simulink model "LBMPC"  (R2018b)
settings: Solver=VariableStepAuto  StartTime=0.0  StopTime=10  RelTol=1e-3
values from neighbouring files (symbols this model uses):
  Ad = expm(A*dT)    [init_ctrl_design.m]    (also in init_ctrl_design_simple.m = eye(2)+A*Ts)
  Bd = (Ad-eye(n))*inv(A)*B    [init_ctrl_design.m]    (also in init_ctrl_design_simple.m = Ts*B)
  beta = 1    [TaylorRemainder.m]    (also in init_ctrl_design.m; init_ctrl_design_simple.m; solveMGCM.m)
  Cd = C    [init_ctrl_design.m]    (also in init_ctrl_design_simple.m = eye(2))
  Dd = D    [init_ctrl_design.m]    (also in init_ctrl_design_simple.m)
  init_cond = [x1-0.35, x2-0.4, x3, 0]    [TaylorRemainder.m]    (also in init_ctrl_design.m; init_ctrl_design_simple.m = [x1-0.35, x2-0.4])
  Ts = 0.01    [APRBSgeneration.m]    (also in draw.m; drawCP.m = 0.1; genTrainingData.m = 0.1; init_ctrl_design.m)
  wn = sqrt(1000)    [TaylorRemainder.m]    (also in init_ctrl_design.m; solveMGCM.m)
  x2_c = 0    [TaylorRemainder.m]    (also in init_ctrl_design.m; init_ctrl_design_simple.m; solveMGCM.m)
  zeta = 1/sqrt(2)    [TaylorRemainder.m]    (also in init_ctrl_design.m)
undefined symbols (not defined in the file or in its folder): DiscIntNeverNeededParam, K
settings Model: Creator=pbevanda  LastModifiedBy=pbevanda

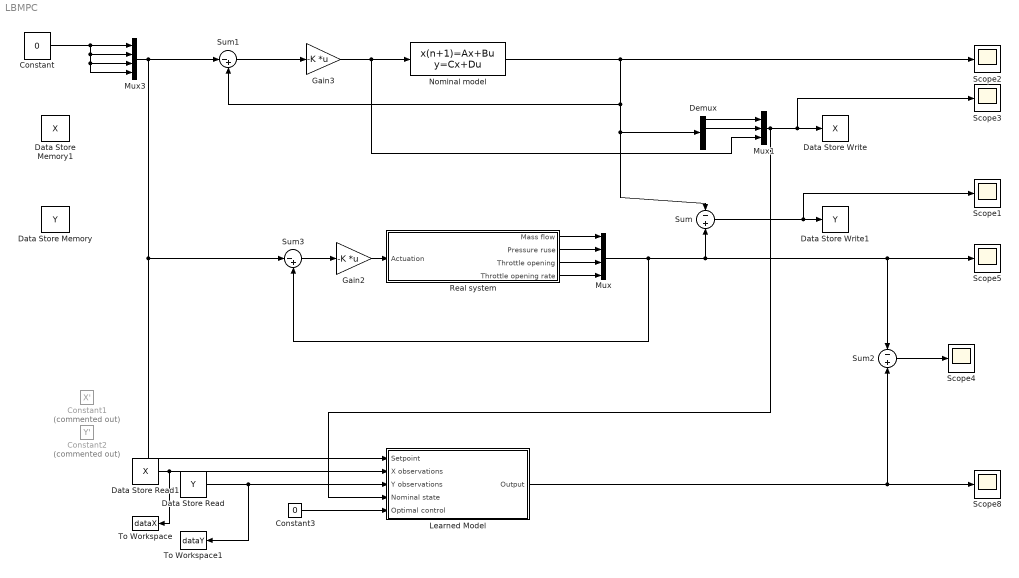
== system LBMPC ==
  "  Nominal model" : DiscreteStateSpace  A=Ad  B=Bd  C=Cd  D=Dd  InitialCondition=init_cond  SampleTime=Ts
  Constant : Constant  Value=0
  Constant1 : Constant  Commented=on  Value=X'  VectorParams1D=off  SampleTime=1
  Constant2 : Constant  Commented=on  Value=Y'  VectorParams1D=off
  Constant3 : Constant  Value=0  VectorParams1D=off
  Data Store Memory : DataStoreMemory  DataStoreName=Y  ReadBeforeWriteMsg=warning  WriteAfterWriteMsg=warning  WriteAfterReadMsg=warning  ShowAdditionalParam=off  OutDataTypeStr=double  Dimensions=4
  Data Store Memory1 : DataStoreMemory  DataStoreName=X  ReadBeforeWriteMsg=warning  WriteAfterWriteMsg=warning  WriteAfterReadMsg=warning  ShowAdditionalParam=off  OutDataTypeStr=double  Dimensions=3
  Data Store Read : DataStoreRead  DataStoreName=Y
  Data Store Read1 : DataStoreRead  DataStoreName=X
  Data Store Write : DataStoreWrite  DataStoreName=X
  Data Store Write1 : DataStoreWrite  DataStoreName=Y
  Demux : Demux
  Gain2 : Gain  Gain=-K  Multiplication=Matrix(K*u)
  Gain3 : Gain  Gain=-K  Multiplication=Matrix(K*u)
  "Learned Model " : Subsystem
  Mux : Mux
  Mux1 : Mux  Inputs=3
  Mux3 : Mux
  Real system : Subsystem
  Scope{1..5,8} (6 alike) : Scope
  Sum : Sum  Inputs=-+
  Sum1 : Sum  Inputs=|-+
  Sum2 : Sum  Inputs=-+
  Sum3 : Sum  Inputs=|-+
  To Workspace : ToWorkspace  VariableName=dataX  SampleTime=-1
  To Workspace1 : ToWorkspace  VariableName=dataY  SampleTime=-1
  wires:
  Gain2/1 -> Real system/1("Actuation ")
  Sum1/1 -> Gain3/1
  Demux/1 -> Mux1/1
  Real system/1("Mass flow ") -> Mux/1
  "  Nominal model"/1 -> Demux/1, Sum/1, Sum1/2, Scope2/1
  Constant/1 -> Mux3/1, Mux3/4, Mux3/3, Mux3/2
  Mux/1 -> Sum3/2, Sum2/1, Scope5/1, Sum/2
  Sum3/1 -> Gain2/1
  Real system/4("Throttle opening rate ") -> Mux/4
  Demux/2 -> Mux1/2
  Mux3/1 -> Sum1/1, "Learned Model "/1(Setpoint), Sum3/1
  Real system/2("Pressure ruse ") -> Mux/2
  Gain3/1 -> "  Nominal model"/1, Mux1/3
  Real system/3("Throttle opening ") -> Mux/3
  Sum/1 -> Scope1/1, Data Store Write1/1
  Constant3/1 -> "Learned Model "/5(Optimal control)
  "Learned Model "/1("Output ") -> Sum2/2, Scope8/1
  Mux1/1 -> "Learned Model "/4(Nominal state), Scope3/1, Data Store Write/1
  Data Store Read/1 -> To Workspace1/1, "Learned Model "/3(Y observations)
  Data Store Read1/1 -> To Workspace/1, "Learned Model "/2("X observations ")
  Sum2/1 -> Scope4/1

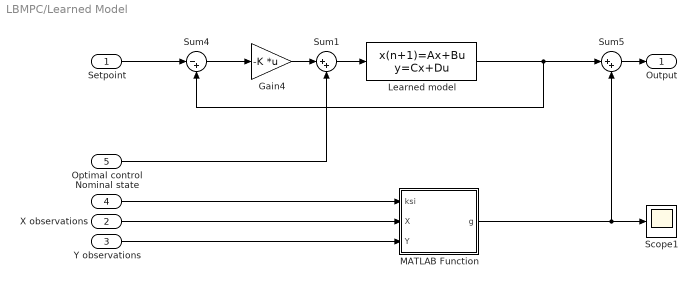
== system LBMPC/Learned Model  ==
  Setpoint : Inport
  "X observations " : Inport  Port=2
  Y observations : Inport  Port=3
  Nominal state : Inport  Port=4
  Optimal control : Inport  Port=5
  Gain4 : Gain  Gain=-K  Multiplication=Matrix(K*u)
  Learned model : DiscreteStateSpace  A=Ad  B=Bd  C=Cd  D=Dd  InitialCondition=init_cond  SampleTime=Ts
  MATLAB Function : MATLAB Function  TreatAsAtomicUnit=on
  Scope1 : Scope
  Sum1 : Sum  Inputs=|++
  Sum4 : Sum  Inputs=|-+
  Sum5 : Sum  Inputs=|++
  "Output " : Outport
  wires:
  Sum4/1 -> Gain4/1
  Learned model/1 -> Sum4/2, Sum5/1
  Setpoint/1 -> Sum4/1
  Y observations/1 -> MATLAB Function/3(Y)
  "X observations "/1 -> MATLAB Function/2(X)
  Nominal state/1 -> MATLAB Function/1(ksi)
  MATLAB Function/1(g) -> Sum5/2, Scope1/1
  Sum5/1 -> "Output "/1
  Sum1/1 -> Learned model/1
  Gain4/1 -> Sum1/1
  Optimal control/1 -> Sum1/2

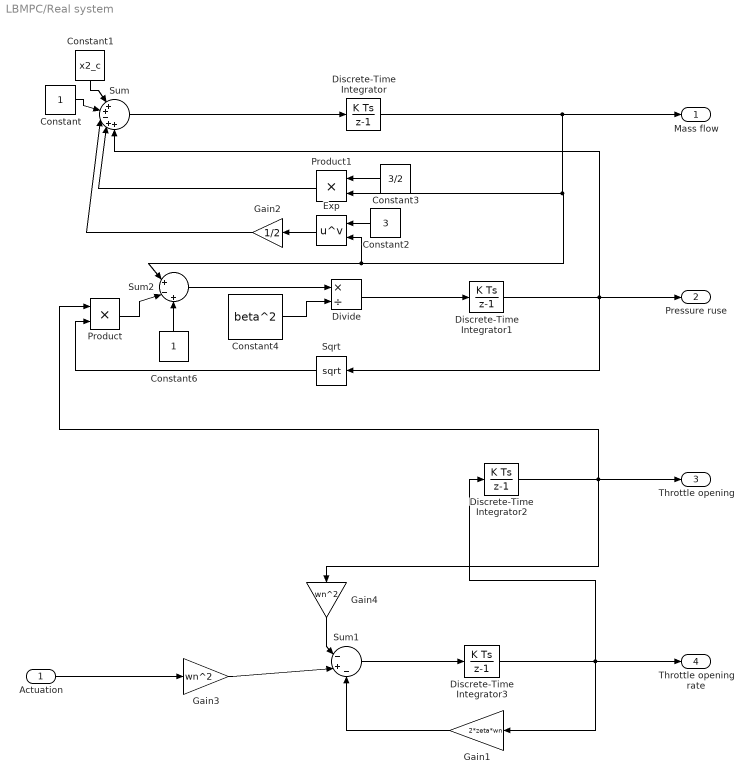
== system LBMPC/Real system ==
  "Actuation " : Inport
  Constant : Constant
  Constant1 : Constant  Value=x2_c
  Constant2 : Constant  Value=3
  Constant3 : Constant  Value=3/2
  Constant4 : Constant  Value=beta^2
  Constant6 : Constant
  Discrete-Time Integrator : DiscreteIntegrator  InitialCondition=init_cond(1)  SampleTime=-1  ICPrevOutput=DiscIntNeverNeededParam  ICPrevScaledInput=DiscIntNeverNeededParam
  Discrete-Time Integrator1 : DiscreteIntegrator  InitialCondition=init_cond(2)  SampleTime=-1  ICPrevOutput=DiscIntNeverNeededParam  ICPrevScaledInput=DiscIntNeverNeededParam
  Discrete-Time Integrator2 : DiscreteIntegrator  InitialCondition=init_cond(3)  SampleTime=-1  ICPrevOutput=DiscIntNeverNeededParam  ICPrevScaledInput=DiscIntNeverNeededParam
  Discrete-Time Integrator3 : DiscreteIntegrator  InitialCondition=init_cond(4)  SampleTime=-1  ICPrevOutput=DiscIntNeverNeededParam  ICPrevScaledInput=DiscIntNeverNeededParam
  Divide : Product  Inputs=*/
  Exp : Math  Operator=pow  SaturateOnIntegerOverflow=on
  Gain1 : Gain  Gain=2*zeta*wn
  Gain2 : Gain  Gain=1/2
  Gain3 : Gain  Gain=wn^2
  Gain4 : Gain  Gain=wn^2
  Product : Product
  Product1 : Product
  Sqrt : Sqrt  SaturateOnIntegerOverflow=on
  Sum : Sum  Inputs=|++-++
  Sum1 : Sum  Inputs=|-+-
  Sum2 : Sum  Inputs=|+-+
  "Mass flow " : Outport
  "Pressure ruse " : Outport  Port=2
  "Throttle opening " : Outport  Port=3
  "Throttle opening rate " : Outport  Port=4
  wires:
  Constant/1 -> Sum/2
  Constant1/1 -> Sum/1
  Constant2/1 -> Exp/1
  Constant4/1 -> Divide/2
  Sum2/1 -> Divide/1
  Constant6/1 -> Sum2/3
  Sqrt/1 -> Product/2
  Product/1 -> Sum2/2
  Divide/1 -> Discrete-Time Integrator1/1
  Exp/1 -> Gain2/1
  Gain2/1 -> Sum/3
  Constant3/1 -> Product1/1
  Product1/1 -> Sum/4
  Sum1/1 -> Discrete-Time Integrator3/1
  Gain1/1 -> Sum1/3
  Gain4/1 -> Sum1/1
  Sum/1 -> Discrete-Time Integrator/1
  Gain3/1 -> Sum1/2
  "Actuation "/1 -> Gain3/1
  Discrete-Time Integrator2/1 -> "Throttle opening "/1, Gain4/1, Product/1
  Discrete-Time Integrator3/1 -> "Throttle opening rate "/1, Discrete-Time Integrator2/1, Gain1/1
  Discrete-Time Integrator/1 -> "Mass flow "/1, Product1/2, Exp/2, Sum2/1
  Discrete-Time Integrator1/1 -> "Pressure ruse "/1, Sum/5, Sqrt/1

== matlab function LBMPC/Learned Model /MATLAB Function ==
  data: g output; ksi input; X input; Y input
function g = oracle(ksi, X, Y)
% g = oracle(ksi, X, Y) performs a nonparametric L2 normalised Nadaraya-Watson kernel regression

bandwidth = 5;  
lambda = 0.1; 
% d = numel(ksi);
s = size(Y,1);
n = size(X,2);

kval = zeros(1,n);
for i=1:n
    kval(i) = exp(-((norm(X(:,i) - ksi).^2)/bandwidth));
end
skval = sum(kval);
weight = kval/(lambda + skval);
y=zeros(s,1);
for i=1:n
    out = weight(i)*Y(:,i);
    y = y + out;
end
g = y;
